simulink model "TestStructure"  (R2023b)
settings: Solver=FixedStepDiscrete  StartTime=0.0  StopTime=inf  FixedStep=SampleTime  RelTol=1e-3
InitFcn:
  | SampleTime = 0.001;
  | ButtonValue=0;
  | load("BusConfig.mat");
undefined symbols (not defined in the file): DiscIntNeverNeededParam
libraries: slrealtimeethercatlib x219, dspfdesign x28, dspstat3 x23, simulink x21, slpidlib x10, dspswit3 x8, commfilt2 x2, dspsigops x1
(part 8 of 8)

== matlab function TestStructure/InterForceControlTask/AO/ColdStartEventGate ==
  data: event_in input; event_out output; t_now input; T_base_default input
function event_out = fcn(event_in, t_now, T_base_default)
%#codegen
% Pass the first AO event immediately, then reject duplicate pulses that
% are too close to the data-derived baseline gait period.
persistent prev seen_first last_accept_t
if isempty(prev)
    prev = false;
    seen_first = false;
    last_accept_t = 0.0;
end

event_out = 0.0;
curr = (event_in ~= 0);
rise = (~prev) && curr;
prev = curr;
if ~rise
    return;
end

T = double(T_base_default);
if ~isfinite(T) || T <= 0.5 || T >= 4.0
    T = 1.66;
end
min_interval = max(0.5, 0.5 * T);
if ~seen_first || (t_now - last_accept_t) >= min_interval
    event_out = 1.0;
    seen_first = true;
    last_accept_t = t_now;
end
end

== matlab function TestStructure/InterForceControlTask/AO/Subsystem1/Abs-based selector/MATLAB Function ==
  data: candidate input; pos_env input; neg_env input; mode output
function mode = select_event_mode(candidate, pos_env, neg_env)
% mode =  1：使用正事件
% mode = -1：使用负事件
% mode =  0：切换时跳过当前目标事件

persistent current_mode pending_mode switching seen_target_event

if isempty(current_mode)
    current_mode = 1;          % 默认用正事件
    pending_mode = 1;
    switching = false;
    seen_target_event = false;
end

% 参数
ratio = 1.2;       % 正负幅值差超过20%才认为该切换
k = 0.4;           % 阈值比例，和你外面的动态阈值保持一致
th_min = 0.05;     % 最小阈值，按你的candidate量级调整

% 根据正负包络得到各自阈值
th_pos = max(k * pos_env, th_min);
th_neg = max(k * neg_env, th_min);

% 默认输出当前模式
mode = current_mode;

% 判断当前应该使用哪个事件方向
desired_mode = current_mode;

if pos_env > ratio * neg_env
    desired_mode = 1;
elseif neg_env > ratio * pos_env
    desired_mode = -1;
end

% 如果发现应该切换：只登记，不立刻切换
if ~switching && desired_mode ~= current_mode
    pending_mode = desired_mode;
    switching = true;
    seen_target_event = false;
end

% 如果正在切换，跳过目标方向的第一个事件脉冲
if switching

    if pending_mode == 1
        target_event = candidate > th_pos;
    else
        target_event = candidate < -th_neg;
    end

    % 目标方向第一个脉冲出现：跳过
    if target_event
        mode = 0;
        seen_target_event = true;
        return;
    end

    % 目标方向第一个脉冲已经结束：正式切换
    if seen_target_event && ~target_event
        current_mode = pending_mode;
        switching = false;
        seen_target_event = false;
        mode = current_mode;
        return;
    end

    % 还没等到目标事件时，继续保持旧模式
    mode = current_mode;
end

== matlab function TestStructure/InterForceControlTask/AO/Subsystem1/If Action Subsystem2/MATLAB Function1 ==
  data: u input; y output; threadhold input
function y = fcn(u, threadhold)
a = mean(u);
b = u - a;
y = (b(end) - b(1))*abs(a)*200;

if abs(y) <= threadhold
    y = 0;
end

== matlab function TestStructure/InterForceControlTask/AO2/MATLAB Function ==
  data: phi input; y output; deltaphi input
function y = fcn(phi,deltaphi)
%#codegen

a = (phi - deltaphi);

if deltaphi<0
    if(a>1)
        a = a-1;
    else
    end
else
    if(a<0)
        a = a+1;
    else
    end
end

y = a;

== matlab function TestStructure/InterForceControlTask/AO/Subsystem1/MATLAB Function ==
  data: y output; u input
function y = Decline_effective(u)
persistent d_start;
persistent d_end;
persistent d_max;

if isempty(d_start)
    d_start = 0;
    d_end = 1;
    d_max = 0;
end

y = 0;

if (u <= d_max * 0.1) && (d_end == 1)
    d_start = 1;
    d_end = 0;
end

if (d_start==1)
    if u < d_max
        y = 1;
        d_start = 0;
    else
        d_max = max(u,d_max);
    end
end

if (d_start == 0)
    if u <= d_max * 0.1
        d_max = 0;
        d_end = 1;
    end
end

== matlab function TestStructure/InterForceControlTask/TorqueController/Subsystem2/MATLAB Function ==
  data: y output; u input
function y = Decline_effective(u)
persistent d_start;
persistent d_end;
persistent d_max;

if isempty(d_start)
    d_start = 0;
    d_end = 1;
    d_max = 0;
end

y = 0;

if (u <= d_max * 0.1) && (d_end == 1)
    d_start = 1;
    d_end = 0;
end

if (d_start==1)
    if u < d_max
        y = 1;
        d_start = 0;
    else
        d_max = max(u,d_max);
    end
end

if (d_start == 0)
    if u <= d_max * 0.1
        d_max = 0;
        d_end = 1;
    end
end

== matlab function TestStructure/InterForceControlTask/AO3/MATLAB Function ==
  data: phi input; y output; deltaphi input
function y = fcn(phi,deltaphi)
%#codegen

a = (phi - deltaphi);

if deltaphi<0
    if(a>1)
        a = a-1;
    else
    end
else
    if(a<0)
        a = a+1;
    else
    end
end

y = a;

== matlab function TestStructure/InterForceControlTask/TorqueController/Subsystem2/If Action Subsystem2/MATLAB Function1 ==
  data: u input; y output; threadhold input
function y = fcn(u, threadhold)
a = mean(u);
b = u - a;
y = (b(end) - b(1))*abs(a)*200;

if abs(y) <= threadhold
    y = 0;
end

== matlab function TestStructure/InterForceControlTask/TorqueController/MATLAB Function3 ==
  data: u input; y output
function y = fcn(u)
    y = (3/(1+exp(-40*(u+(1/10))))-3)+(3/(1+exp(-40*(u-(1/10)))));
end

== matlab function TestStructure/InterForceControlTask/AO/Subsystem1/Detector1/VoltageToFootLoad ==
  data: p8 input; leftLoad output; rightLoad output
function [leftLoad, rightLoad] = VoltageToFootLoad(p8)
%#codegen
p = double(p8(:));

% The selected channels use a stable unloaded voltage across sessions.
% A fixed baseline avoids false events while a cold-start maximum settles.
baseline = 2.6 * ones(8,1);
leftIdx = int32([2 3]);
rightIdx = int32([6 7]);

load = max(baseline - p, 0.0);
for n = 1:2
    k = leftIdx(n);
    if ~isfinite(p(k)) || p(k) <= 0.1
        load(k) = 0.0;
    end
    k = rightIdx(n);
    if ~isfinite(p(k)) || p(k) <= 0.1
        load(k) = 0.0;
    end
end

leftLoad = sum(load(leftIdx));
rightLoad = sum(load(rightIdx));
end

== matlab function TestStructure/InterForceControlTask/DMP/MATLAB Function6 ==
  data: weights output; p_resampled_in input; centers output; widths output; y0 output; v0 output; goal output; segment_len input; A_demo output; y0_demo output; StartEvent input; ComputeEnable input; alpha_z input; alpha_x input; progress output; ChunkSize input; done output
function [weights, centers, widths, y0, v0, goal, A_demo, y0_demo, progress, done] = ...
    learn_from_trajectory_incremental( ...
        p_resampled_in, segment_len, StartEvent, ComputeEnable, ...
        alpha_z, alpha_x, ChunkSize)
%#codegen

% —— 统一成 double，避免上游给到单/整型 —— 
% p_resampled_in = double(p_resampled_in);
% segment_len    = double(segment_len);
% StartEvent     = double(StartEvent);
% ComputeEnable  = double(ComputeEnable);
% alpha_z        = double(alpha_z);
% alpha_x        = double(alpha_x);
% ChunkSize      = double(ChunkSize);

% —— 常量 —— 
n_bfs  = 400;
tau    = 1.0;
beta_z = alpha_z / 4.0;

% —— 持久变量（全部提前声明并默认初始化）——
persistent L idx dt_norm ...
           y0_demo_t A_demo_t y0_t v0_t goal_t ...
           centers_t widths_t ...
           num_t den_t ...
           prev_y prev_v inited ...
           p_norm_t demo_v_t demo_a_t

if isempty(inited)
    % 初始默认（保证任何路径下都有定义）
    inited     = false;
    L          = 1;
    idx        = 1;
    dt_norm    = 1.0;
    y0_demo_t  = 0.0;
    A_demo_t   = 1.0;
    y0_t       = 0.0;
    v0_t       = 0.0;
    goal_t     = 0.0;
    centers_t  = zeros(1, n_bfs);
    widths_t   = ones(1, n_bfs);
    num_t      = zeros(1, n_bfs);
    den_t      = zeros(1, n_bfs);
    prev_y     = 0.0;
    prev_v     = 0.0;
    p_norm_t   = 0.0;
    demo_v_t   = 0.0;
    demo_a_t   = 0.0;
end

% —— 输出缺省值（即使未开始也有稳定输出）——
weights  = zeros(1, n_bfs);
centers  = centers_t;
widths   = widths_t;
y0       = y0_t;
v0       = v0_t;
goal     = goal_t;
A_demo   = A_demo_t;
y0_demo  = y0_demo_t;
progress = 0.0;
done     = 0.0;

% ====== 若 StartEvent 触发：初始化一轮增量学习 ======
if (StartEvent ~= 0) && (segment_len >= 2)
    L = max(1, floor(segment_len));          % 防御性：整数长度
    % 幅值统计（整段一次，代价极小）
    % y0_demo_t = p_resampled_in(1);
    pmax = max(p_resampled_in(1:L));
    pmin = min(p_resampled_in(1:L));
    %y0_demo由pmin替代
    y0_demo_t = pmin;
    A_demo_t = pmax - pmin;
    if A_demo_t < 1e-8, A_demo_t = 1.0; end
    
    p_norm_t  = (p_resampled_in(1:L) - pmin) / A_demo_t;
    y0_t   = p_norm_t(1);
    goal_t = p_norm_t(L);

    dt_norm = tau / max(1, (L - 1));
    if L >= 2
        demo_v_t       = [ (p_norm_t(2)-p_norm_t(1))/dt_norm ; diff(p_norm_t)./dt_norm ];
        demo_a_t       = [ (demo_v_t(2)-demo_v_t(1))/dt_norm ; diff(demo_v_t)./dt_norm ];
        v0_t           = demo_v_t(1);
    else
        demo_v_t = 0.0;  demo_a_t = 0.0;  v0_t = 0.0;
    end
    
    % 基函数网格
    % ext = 4;
    cc  = exp(-alpha_x * linspace(0, 1, n_bfs));
    ww  = n_bfs^2 ./ cc;
    centers_t = cc;
    widths_t  = ww;

    % % 基函数网格（首尾各裁4）
    % ext = 4;
    % cc  = exp(-alpha_x * linspace(0, 1, n_bfs + 2*ext));
    % ww  = (n_bfs + 2*ext)^2 ./ cc;
    % centers_t = cc((1+ext):(end-ext));
    % widths_t  = ww((1+ext):(end-ext));

    % 累加器清零与指针
    num_t = zeros(1, n_bfs);
    den_t = zeros(1, n_bfs);
    idx   = 1;
    prev_y = y0_t; 
    prev_v = v0_t;

    inited = true;
end

% —— 若尚未开始（没收到 StartEvent），直接返回缺省输出 —— 
if ~inited
    return;
end

% ====== 1ms Tick：每次吃 ChunkSize 个样本 ======
if (ComputeEnable ~= 0) && (idx <= L)
    % 夹紧 ChunkSize 合理范围
    cs = min( max(1, floor(ChunkSize)), L - idx + 1 );

    for k = 0:(cs-1)
        j  = idx + k;                      % 第 j 个样本（1-based）

        % —— 用持久的预计算序列 —— 
        yj = p_norm_t(j);
        vj = demo_v_t(j);
        aj = demo_a_t(j);

        prev_y = yj; 
        prev_v = vj;

        % 规范时间与门控
        tj = (j - 1) * dt_norm;
        sj = exp(-alpha_x * tj);

        % f_target（知乎改进方案）
        f_target = ( tau*tau*aj - alpha_z*(beta_z*(goal_t - yj) - tau*vj) )/alpha_z ...
                   + sj*(goal_t - y0_t);
        % f_target = ( tau*tau*aj - alpha_z*(beta_z*(goal_t - yj) - tau*vj) )/alpha_z;

        % 累加充要统计量
        psi_row = exp( - widths_t .* (sj - centers_t).^2 );
        num_t   = num_t + (sj * f_target) * psi_row;
        den_t   = den_t + (sj*sj) * psi_row;
    end
    idx = idx + cs;
end

% —— 进度条 —— 
progress = min(1.0, idx / max(1, L));

% ====== 全段完成：输出权重并置 done ======
if idx > L
    weights = num_t ./ (den_t + 1e-12);
    centers = centers_t;
    widths  = widths_t;
    y0      = y0_t;
    v0      = v0_t;
    goal    = goal_t;
    A_demo  = A_demo_t;
    y0_demo = y0_demo_t;

    done    = 1.0;
    % 如需下一次 StartEvent 重新开始，可在此处选择：
    % inited = false;
end
end

== matlab function TestStructure/InterForceControlTask/AO2/Select/MATLAB Function1 ==
  data: u input; y output
function y = fcn(u)
    y = (3/(1+exp(-40*(u+(1/10))))-3)+(3/(1+exp(-40*(u-(1/10)))));
end

== matlab function TestStructure/InterForceControlTask/AO2/Subsystem/Subsystem/MATLAB Function ==
  data: phi input; y output; deltaphi input
function y = fcn(phi,deltaphi)
%#codegen

a = floor(phi/(2*pi));

y = (phi - a*2*pi -deltaphi*pi);

== matlab function TestStructure/InterForceControlTask/AO2/Subsystem/Subsystem1/MATLAB Function ==
  data: phi input; y output; deltaphi input
function y = fcn(phi,deltaphi)
%#codegen

a = floor(phi/(2*pi));

y = (phi - a*2*pi -deltaphi*pi);

== matlab function TestStructure/InterForceControlTask/AO2/Subsystem/Subsystem3/MATLAB Function ==
  data: phi input; y output; deltaphi input
function y = fcn(phi,deltaphi)
%#codegen

a = floor(phi/(2*pi));

y = (phi - a*2*pi -deltaphi*pi);

== matlab function TestStructure/InterForceControlTask/AO2/Subsystem/Subsystem5/MATLAB Function ==
  data: phi input; y output; deltaphi input
function y = fcn(phi,deltaphi)
%#codegen

a = floor(phi/(2*pi));

y = (phi - a*2*pi -deltaphi*pi);

== matlab function TestStructure/InterForceControlTask/DMP/MATLAB Function8 ==
  data: FastStartEvent input; weights input; centers input; widths input; y0 input size=[1 1]; v0 input; goal input size=[1 1]; A_demo input size=[1 1]; y0_demo input size=[1 1]; alpha_z input; alpha_x input; TriggerEvent input; s input size=[1 1]; dt input size=[1 1]; tau input size=[1 1]; y_real output; Amplitude input; HoldRatio input; HoldRefSec input; v_real output; right_start_real input; playback_phi output
function [y_real,v_real,playback_phi] = trajectory_generator( ...
    FastStartEvent, weights, centers, widths, y0, v0, goal, A_demo, y0_demo, ...
    alpha_z, alpha_x, TriggerEvent, s, dt, tau, Amplitude, ...
    HoldRatio, HoldRefSec, right_start_real )
% 生成端（残差版）：支持 tau 时间缩放 + 完成后 hold + min–max 反归一化
% 输入 s：这里把它当作 AO 的“相位”Phi∈[0,1] 来用（线性锯齿即可）
% 输出 y_real：反归一化后的轨迹（y*A_demo + pmin），其中 y0_demo 端口承载 pmin
%#codegen

% --- 常量 ---
beta_z = alpha_z / 4.0;
SAFE_CENTER = 0.0;   % 不稳定时希望缓慢回到的"安全角度"，单位与 y_real 一致，可改
SAFE_BAND   = 0.0;   % 认为"已经够安全”的带宽，比如 ±5 度内就直接原地 hold
ENABLE_STABLE_GATE = false;   % true=启用稳定门，false=关闭稳定门

% --- 持久状态（内部 y, y_dot；相位缩放用的内部进度 u；完成标志） ---
persistent y y_dot u phi_prev inited trig_prev fast_prev fast_seen_count dmp_ready_for_start started pending_reset just_started first_playback_protected
persistent hold_ticks hold_active
persistent delay_ticks delay_active prev_y_real prev_v_real refrac_ticks prestart_hold prestart_hold_valid  
persistent A_prev y0d_prev
persistent g_tAcc g_buf g_has g_outOK g_safeY

if isempty(refrac_ticks), refrac_ticks = 0; end
if isempty(fast_prev), fast_prev = 0.0; end
if isempty(fast_seen_count), fast_seen_count = int32(0); end
if isempty(dmp_ready_for_start), dmp_ready_for_start = 0.0; end
if isempty(first_playback_protected), first_playback_protected = false; end
if isempty(A_prev),   A_prev   = A_demo; end
if isempty(y0d_prev), y0d_prev = y0_demo; end



if isempty(prev_y_real), prev_y_real = 0; end
if isempty(prestart_hold), prestart_hold = 0.0; end
if isempty(prestart_hold_valid), prestart_hold_valid = false; end
if isempty(prev_v_real), prev_v_real = 0; end

if isempty(inited)
    first_cycle = true;
    y = y0;
    y_dot = v0;
    u = 0;  
    phi_prev = 0;
    finished = false;
    trig_prev = false;
    inited = true;
    started = false;
    pending_reset = false;   % 新增：检测到开始沿后，下一帧再复位
    just_started  = false;   % 新增：复位后的首帧只打起点，不推进
    y0_latch = y0; v0_latch = v0; goal_latch = goal;   % 参数锁存（用于握手）
    hold_ticks = 0;
    hold_active = false;
    delay_ticks = 0;
    delay_active = false;
    eps_param = 1e-6;
    g_tAcc = 0.0;              % 距上次沿累计的时间
    g_buf  = [Inf Inf Inf];    % 最近3个周期（秒）
    g_has  = 0;                % 已记录周期数(<=3)
    g_outOK = ~ENABLE_STABLE_GATE;           % 是否允许输出
    g_safeY = 0.0;              % 不稳定时要渐近回到的安全位(这里取0)
end

playback_phi = u;
y_real = prev_y_real;   % 默认保持上一帧
v_real = prev_v_real;

% --- 相位增量（把第 11 个输入 s 当作相位 Phi）---
Phi = s;
raw_dphi = Phi - phi_prev;   % 保留原始差分用于回绕沿判定
dphi = raw_dphi;
% 处理 1→0 回绕；防止偶发负跳
if dphi < -0.5
    dphi = (1 - phi_prev) + Phi;
elseif dphi < 0
    dphi = 0;
end
wrap_edge = (raw_dphi < -0.5);  % 新增：相位 1->0 回绕沿
phi_prev = Phi;

% --- Phase0Event 上升沿检测 ---
trig_edge = false;

if (trig_prev == false && TriggerEvent == true)
    trig_edge = true;
end
trig_prev = TriggerEvent;

fast_curr = (FastStartEvent ~= 0);
fast_edge_raw = ((fast_prev == 0.0) && fast_curr);
fast_prev = double(fast_curr);
fast_edge = fast_edge_raw;
if fast_edge_raw
    fast_seen_count = fast_seen_count + 1;
end

% ===== 稳定门：用 TriggerEvent 的上升沿统计周期 =====
if ENABLE_STABLE_GATE
    % 累计时间
    g_tAcc = g_tAcc + dt;

    if trig_edge
        T = g_tAcc;         % 一个完整周期（秒）
        g_tAcc = 0.0;

        % 只保留最近3个周期
        g_buf = [g_buf(2:3) T];
        g_has = min(g_has + 1, 3);

        % 判稳：max-min <= max(绝对阈, 相对阈*均值)
        if g_has >= 3
            Tmean   = (g_buf(1)+g_buf(2)+g_buf(3))/3;
            Tspan   = max(g_buf) - min(g_buf);
            TOL_REL = 0.40;
            TOL_ABS = 0.20;
            g_outOK = (Tspan <= max(TOL_ABS, TOL_REL*Tmean));
        else
            g_outOK = false;
        end
    end
else
    g_outOK = true;
end
% ===== 稳定门 END =====


% ---------- DMP ready 前：不推进、不积分，输出当前右腿位置 ----------
if ~started
    % The first FastStart already means one complete trajectory window
    % has been learned. Take over immediately at this boundary.
    start_edge = fast_edge;
else
    start_edge = false;
    if trig_edge
        start_edge = true;
    end
end

if ~started
    if start_edge
        started = true;
        first_playback_protected = true;
        dmp_ready_for_start = 0.0;
        first_cycle = false;
        pending_reset = false;
        just_started = false;
        y0_latch = y0; v0_latch = v0; goal_latch = goal;
        A_seed = sign(A_demo) * max(abs(A_demo), 1e-9);


        y = (right_start_real - y0_demo) / A_seed;
        y_dot = 0;
        u = 0;
        finished = false;
        A_prev = A_seed;
        y0d_prev = y0_demo;
        y_real = right_start_real;
        v_real = 0;
        prev_y_real = y_real;
        prev_v_real = v_real;
        g_safeY = y_real;
        return;
    else
        y_real = right_start_real;
        v_real = 0;
        prev_y_real = y_real;
        prev_v_real = v_real;
        g_safeY = y_real;
        return;
    end
end
% ---------- 以上仅影响“第一拍开始前/开始当拍”；之后流程不变 ----------

% ---- 开始后的第1帧：真正用已更新的 y0/v0 执行复位，并返回 ----
if pending_reset

    % ====== 软复位 + 坐标重投影（无跳变、无扭动）======
    % 新一拍的仿射参数（可能刚换）
    A_new   = A_demo;
    y0_new  = y0_demo;

    % 防除零
    A_new = sign(A_new) * max(abs(A_new), 1e-9);
    A_prev = sign(A_prev) * max(abs(A_prev), 1e-9);

    % 1) 位置连续：把内部 y 重写为“在新坐标下仍等于上一帧输出”的值
    %    令 y_new 满足：prev_y_real = y_new * A_new + y0_new
    y = (prev_y_real - y0_new) / A_new;

    % 2) 速度连续（可选但强烈建议）：让 y_real_dot 连续
    %    之前：y_real_dot_prev = y_dot * A_prev
    %    之后：y_real_dot_now  = y_dot_new * A_new  → 令两者相等
    y_dot = y_dot * (A_prev / A_new);

    % 3) 开启新拍：只把进度清零，其它状态保持
    u             = 0;
    finished      = false;
    pending_reset = false;

    % 4) 更新“上一拍参数”备下次用
    A_prev   = A_new;
    y0d_prev = y0_new;

    % % 5) 当帧输出保持不变（绝对连续）
    % y_real      = prev_y_real;
    % prev_y_real = y_real;
    % v_real = prev_v_real;
    % prev_v_real = v_real;
    % return;

end

% ---- 开始后的第2帧：只输出起点，不推进、不积分 ----
if just_started
    y_real = y0 * A_demo + y0_demo;

    % ---- 稳定器输出门控 + 回到0附近 ----
    if g_outOK
        % 稳定：直接用 DMP 输出，并同步安全位
        g_safeY = y_real;
    else
        % 不稳定：不跟 DMP，缓慢回到0附近
        T_back = 0.3;                         % 回零时间常数(秒)，可调
        alpha  = dt / max(T_back, 1e-3);
        if alpha > 1, alpha = 1; end
        if abs(g_safeY - SAFE_CENTER) <= SAFE_BAND
            % 已在安全带内：直接 hold，不再往 SAFE_CENTER 拉
            y_real = g_safeY;
        else
            % 不在安全带：缓慢向 SAFE_CENTER 收敛
            g_safeY = g_safeY + alpha * (SAFE_CENTER - g_safeY);
            y_real  = g_safeY;
        end
    end
    v_real      = 0;
    prev_y_real = y_real;  % 保证后续复位/重投影的连续性
    prev_v_real = v_real;
    return;
end


% === 新增：首播 hold 段（保持 y0，冻结积分与u推进）===
if hold_active
    if hold_ticks > 0
        hold_ticks = hold_ticks - 1;
        % 输出固定起点；不更新 u / y_dot / y
        y_real = y * A_demo + y0_demo;
        v_real = y_dot * A_demo;
        prev_v_real = v_real;
        return;
    else
        hold_active = false;    % hold 结束，开始正常推进
        end
end

% 是否允许未完成就抢占（true=保持原行为；false=等当前拍走完）
allow_preempt = true;  % 建议设 false 来保幅值/保形状

if (trig_edge && refrac_ticks==0)
    if allow_preempt || (u >= 1 - 1e-6)
        % 允许抢占，或当前拍已完成：照常进入延迟/复位流程

        delay_ticks  = max(0, round((HoldRatio * HoldRefSec) / max(dt,1e-6)));
        delay_active = (delay_ticks > 0);
        pending_reset = true; 
        finished = false; 
        first_cycle = false;
        refrac_ticks  = round(0.02 / max(dt,1e-6));
        % if delay_active
        %     y_real = prev_y_real; 
        %     prev_y_real = y_real; 
        %     v_real = 0;
        %     prev_v_real = v_real;
        %     return;
        % else
        %     pending_reset = true; 
        %     y_real = prev_y_real; 
        %     prev_y_real = y_real; 
        %     v_real = 0;
        %     prev_v_real = v_real;
        %     return;
        % end
    else
        % 不允许抢占且未完成：忽略这次触发，继续把当前拍播完
        % （也可以在这里置一个 overrun 标志供你观察）
        % y_real 默认已经是 prev_y_real；继续向下正常生成
    end
end


% === 延迟阶段：保持上一拍末值，直到 delay_ticks 归零 ===
if delay_active
    if delay_ticks > 0
        delay_ticks = delay_ticks - 1;
        y_real       = prev_y_real;
        v_real       = prev_v_real;
        prev_y_real  = y_real;
        prev_v_real  = v_real;
        return;
    else
        delay_active = false;
        % pending_reset = true;                          % 标记下一帧在 pending_reset 中复位
        % y_real = prev_y_real;                          % 这一帧仍保持末值
        % v_real = 0;
        % prev_v_real = v_real;
        % return;
    end
end

% ====== 拍中参数变化的“连续重投影”（无跳变、无扭动）======
% 任何时候只要 A_demo 或 y0_demo 发生明显变化，就把内部 y/y_dot
% 映射到新坐标，使 y_real 与其导数连续，再继续积分。
eps_aff = 1e-9;  % 防除零
A_now   = sign(A_demo) * max(abs(A_demo), eps_aff);
A_old   = sign(A_prev) * max(abs(A_prev), eps_aff);

if (abs(A_now - A_prev) > 1e-6) || (abs(y0_demo - y0d_prev) > 1e-6)
    % 1) 位置连续：令 y_new 满足 prev_y_real = y_new*A_now + y0_demo
    y = (prev_y_real - y0_demo) / A_now;

    % 2) 速度连续：y_real_dot 旧= y_dot*A_old，新= y_dot_new*A_now → 相等
    y_dot = y_dot * (A_old / A_now);

    % 3) 更新“上一帧参数”
    A_prev   = A_now;
    y0d_prev = y0_demo;

    % 4) 当帧保持输出（绝对连续），下一帧再按新坐标继续积分
    y_real      = prev_y_real;
    prev_y_real = y_real;
    v_real = prev_v_real;
    prev_v_real = v_real;
    return;
end




% --- 内部进度按 tau 缩放推进（时间放缩）---
u = u + dt / max(tau, 1e-6);     % standard DMP scaling; delayed events only prevent early reset
if u > 1
    u = 1;
elseif u < 0
    u = 0;
end

% --- 若已完成：强制 hold 在终点并直接反归一化输出 ---
if u >= 1 - 1e-6
    first_playback_protected = false;
    finished = true;

    % 当前 DMP 的“原始”位置/速度
    y_dmp = y * A_demo + y0_demo;
    v_dmp = A_demo * y_dot;

    if g_outOK
        % —— 稳定：直接跟随 DMP —— 
        y_real  = y_dmp;
        v_real  = v_dmp;
        g_safeY = y_real;
    else
        % —— 不稳定：按 SAFE_CENTER 慢慢回零，同时给出和该轨迹一致的速度 —— 
        T_back = 0.3;
        alpha  = dt / max(T_back, 1e-3);
        if alpha > 1, alpha = 1; end

        if abs(g_safeY - SAFE_CENTER) <= SAFE_BAND
            % 已在安全带内：原地 hold
            y_new = g_safeY;
        else
            % 不在安全带：缓慢向 SAFE_CENTER 收敛
            g_safeY = g_safeY + alpha * (SAFE_CENTER - g_safeY);
            y_new  = g_safeY;
        end

        y_real = y_new;
        % 用输出位置的一阶差分作为“安全”的参考速度
        v_real = (y_new - prev_y_real) / max(dt, 1e-6);
    end

    prev_y_real = y_real;
    prev_v_real = v_real;
    return;
end


% --- 门控/相位：与学习端保持一致（线性或指数二选一） ---
% 线性门控（推荐）：ss 从 1→0
% ss = 1 - u;
% if ss < 1e-6, ss = 1e-6; end

% 指数门控
ss = exp(-alpha_x * u);

% --- 基函数响应（在 s 空间计算；此处用 ss 作为 s）---
psi = exp( - widths .* (ss - centers).^2 );
den = sum(psi) + 1e-12;
if den == 0
    % 极端数值保护
    psi(1) = 1; den = 1;
end
f_shape = (psi * weights.') / den;

% 残差版：f 再乘 s（=ss），仅拟合“形状残差”
f = f_shape * ss;

% --- 动力学（残差版配对：保留 -alpha_z*ss*(goal-y0)）---
y_ddot = ( alpha_z*(beta_z*(goal - y) - tau*y_dot) ...
           + alpha_z * f * Amplitude ...
           - alpha_z * ss * (goal - y0) ) / (tau^2);

% --- 数值积分 ---
y_dot = y_dot + dt * y_ddot;
y     = y     + dt * y_dot;

% --- 反归一化（学习端为 min–max：p_norm=(p - pmin)/A_demo）---
% 因此生成端对应 y_real = y*A_demo + pmin；这里 y0_demo 端口承载 pmin

y_real = y * A_demo + y0_demo;
v_real = A_demo * y_dot;

% --- 反归一化后，先保存 DMP 的“原始”位置和速度 ---
y_dmp = y * A_demo + y0_demo;
v_dmp = A_demo * y_dot;

if g_outOK
    % ======= 稳定：直接用 DMP 的位置和速度 =======
    y_real  = y_dmp;
    v_real  = v_dmp;
    g_safeY = y_real;
else
    % ======= 不稳定：只跟稳定器的缓慢回零轨迹 =======
    T_back = 0.3;                            
    alpha  = dt / max(T_back, 1e-3);
    if alpha > 1, alpha = 1; end

    if abs(g_safeY - SAFE_CENTER) <= SAFE_BAND
        % 已在安全带内：原地 hold
        y_new = g_safeY;
    else
        % 不在安全带：缓慢向 SAFE_CENTER 收敛
        g_safeY = g_safeY + alpha * (SAFE_CENTER - g_safeY);
        y_new  = g_safeY;
    end

    y_real = y_new;
    % 用稳定器轨迹的一阶差分当作参考速度
    v_real = (y_new - prev_y_real) / max(dt, 1e-6);
end

prev_y_real = y_real;
prev_v_real = v_real;


if refrac_ticks > 0
    refrac_ticks = refrac_ticks - 1;
end
end

== matlab function TestStructure/InterForceControlTask/DMP/Phase_shifter ==
  data: Phase0Event_H input; t_ref output; t_now input; T_base_default input
function t_ref = DelayAfterTwoEvents_tref(Phase0Event_H, t_now, T_base_default)
%#codegen
% The data-derived default is active immediately. After three measured
% raw AO periods, switch to the rolling three-period average.
persistent prev seen_first t_prev T1 T2 T3 measured_count t_ref_last
if isempty(prev)
    default_T = sanitizePeriod(T_base_default);
    prev = false;
    seen_first = false;
    t_prev = 0.0;
    T1 = default_T;
    T2 = default_T;
    T3 = default_T;
    measured_count = int32(0);
    t_ref_last = default_T;
end

t_ref = t_ref_last;
curr = (Phase0Event_H ~= 0);
rise = (~prev) && curr;
prev = curr;

if rise
    if ~seen_first
        seen_first = true;
        t_prev = t_now;
    else
        dt = t_now - t_prev;
        if isfinite(dt) && dt > 0.5 && dt < 4.0
            T3 = T2;
            T2 = T1;
            T1 = dt;
            measured_count = measured_count + 1;
            if measured_count >= 3
                t_ref_last = (T1 + T2 + T3) / 3.0;
            end
        end
        t_prev = t_now;
    end
end
t_ref = t_ref_last;
end

function T = sanitizePeriod(value)
T = double(value);
if ~isfinite(T) || T <= 0.5 || T >= 4.0
    T = 1.66;
end
end

== matlab function TestStructure/InterForceControlTask/DMP/Subsystem/DelaySamplesFromPrev ==
  data: t_prev input; ratio input; N output; dt input
function N = DelaySamplesFromPrev(t_prev, ratio, dt)
%#codegen
% 按上一拍周期 t_prev 和当前 ratio 计算整数采样延迟，
% 但一拍内保持不变

persistent N_hold t_prev_last inited
if isempty(inited)
    inited     = false;
    N_hold     = int32(0);
    t_prev_last= 0.0;
end

dt    = max(dt,1e-6);
t_prev= max(t_prev,5*dt);
ratio = max(ratio,0.0);

%  只在检测到 t_prev 发生变化时，更新一次 N_hold
%   （即：每次 AO 识别到新的周期，才换一个延迟）
if ~inited || abs(t_prev - t_prev_last) > 0.5*dt
    Nd        = round((ratio * t_prev) / dt);    % 整数采样
    N_hold    = int32(max(0, Nd));
    t_prev_last = t_prev;
    inited    = true;
end

% 一拍内输出始终为 N_hold（ratio 中途再变也不影响当前拍）
N = N_hold;

== matlab function TestStructure/InterForceControlTask/DMP/Subsystem/EventDelay ==
  data: trig_in input; N input; out output; tau input
function out = PhaseEventDelay_ScaledIntervals(trig_in, N, tau)
%#codegen
% N is valid from cold startup because Phase_shifter starts from the
% data-derived baseline. Queue the first delayed candidate immediately.
MAX_QUEUE = int32(128);
persistent prev sample_idx last_candidate have_candidate scaled_target
persistent queue head tail count
if isempty(prev)
    prev = false;
    sample_idx = int64(0);
    last_candidate = int64(0);
    have_candidate = false;
    scaled_target = int64(0);
    queue = zeros(1, 128, 'int64');
    head = int32(1);
    tail = int32(1);
    count = int32(0);
end

tau = max(double(tau), 1e-6);
out = false;
curr = (trig_in ~= 0);
edge = (~prev) && curr;
prev = curr;

if edge
    candidate = sample_idx + int64(max(0, round(double(N))));
    if ~have_candidate
        scaled_target = candidate;
        have_candidate = true;
    else
        candidate_period = candidate - last_candidate;
        if candidate_period > 0
            scaled_target = scaled_target + int64(max(1, round(tau * double(candidate_period))));
        end
    end
    last_candidate = candidate;

    if scaled_target > 0 && count < MAX_QUEUE
        queue(tail) = scaled_target;
        tail = tail + 1;
        if tail > MAX_QUEUE, tail = int32(1); end
        count = count + 1;
    end
end

if count > 0 && sample_idx >= queue(head)
    out = true;
    head = head + 1;
    if head > MAX_QUEUE, head = int32(1); end
    count = count - 1;
end
sample_idx = sample_idx + 1;
end

== matlab function TestStructure/InterForceControlTask/AO1/MATLAB Function ==
  data: phi input; y output; deltaphi input
function y = fcn(phi,deltaphi)
%#codegen

a = (phi - deltaphi);

if deltaphi<0
    if(a>1)
        a = a-1;
    else
    end
else
    if(a<0)
        a = a+1;
    else
    end
end

y = a;

== matlab function TestStructure/InterForceControlTask/DMP/Subsystem/PhiOmega_DelayRebuild ==
  data: event_delay input; dt_sec input; phi_delay output; omega_delay output; T_base_default input
function [phi_delay, omega_delay] = RebuildPhiOmegaFromDelayedEvent(event_delay, dt_sec, T_base_default)
%#codegen
% Diagnostic delayed-event phase. Hold the shared default until three
% complete delayed periods exist.
persistent prev_evt t_since T1 T2 T3 T_avg measured_count seen_first
if isempty(prev_evt)
    default_T = sanitizePeriod(T_base_default);
    prev_evt = false;
    t_since = 0.0;
    T1 = default_T;
    T2 = default_T;
    T3 = default_T;
    T_avg = default_T;
    measured_count = int32(0);
    seen_first = false;
end

dt_sec = max(dt_sec, 1e-6);
curr = (event_delay ~= 0);
rise = (~prev_evt) && curr;
prev_evt = curr;
t_since = t_since + dt_sec;

if rise
    if seen_first
        last_period = t_since;
        if isfinite(last_period) && last_period > 0.5 && last_period < 6.0
            T3 = T2;
            T2 = T1;
            T1 = last_period;
            measured_count = measured_count + 1;
            if measured_count >= 3
                T_avg = (T1 + T2 + T3) / 3.0;
            end
        end
    else
        seen_first = true;
    end
    t_since = 0.0;
end

omega_delay = 1.0 / max(T_avg, 0.1);
phi_delay = min(max(t_since * omega_delay, 0.0), 1.0);
end

function T = sanitizePeriod(value)
T = double(value);
if ~isfinite(T) || T <= 0.5 || T >= 4.0
    T = 1.66;
end
end

== matlab function TestStructure/InterForceControlTask/DMP/compute_chunk ==
  data: segment_len input; cs output; T_prev input; tick_s input
function cs = compute_chunk(segment_len, T_prev, tick_s)
%#codegen
% 计算每个1ms tick应处理的样本数（ChunkSize）
% 保证输出 cs 为 double，避免 uint16 → double 的隐式写入错误

% 明确输出类型（初始化一次即可设定为 double）
cs = 0.0;

% 转 double，防止上游给了 uint16/int
segment_len_d = double(segment_len);
T_prev_d      = double(T_prev);
tick_d        = double(tick_s);

% 防御性处理
if ~(isfinite(segment_len_d) && segment_len_d > 0)
    segment_len_d = 1.0;
end
if ~(isfinite(T_prev_d) && T_prev_d > 0)
    % 第一拍没有上一周期长度时给个保守默认
    T_prev_d = 0.8;   % 例如默认0.8s步期，可按需修改
end
tick_d = max(tick_d, 1e-6);

% 计算 M 和 ChunkSize
M  = max(1.0, round(T_prev_d / tick_d));
cs = ceil(segment_len_d / M);
cs = min(max(cs, 1.0), segment_len_d);
end

== matlab function TestStructure/InterForceControlTask/DMP/compute_chunk2 ==
  data: phase_edge input; N_available output; start_edge input; compute_tick input; done input; N_used output; Slack output
function [N_available, N_used, Slack] = tick_counters(phase_edge, start_edge, compute_tick, done)
%#codegen
persistent cnt_cycle cnt_used latched_used have_used
if isempty(cnt_cycle)
    cnt_cycle = 0; cnt_used = 0; latched_used = 0; have_used = false;
end

% 周期计数：Phase0Event 上升沿复位
if phase_edge ~= 0
    N_available = cnt_cycle;     % 上一拍统计值
    Slack       = max(0, N_available - latched_used);
    cnt_cycle   = 0;             % 开始新一拍
else
    N_available = -1;            % 非更新时刻可输出 -1 或保持上次外部 Sample&Hold
    Slack       = -1;
end

% 一拍内的 10ms 窗口统计
if compute_tick ~= 0
    cnt_cycle = cnt_cycle + 1;
end

% 学习用的 10ms 计数：从 start_edge 后开始累加，直到 done
if start_edge ~= 0
    cnt_used = 0; have_used = false;
end
if (compute_tick ~= 0) && (done == 0)
    cnt_used = cnt_used + 1;
end
if (done ~= 0) && ~have_used
    latched_used = cnt_used;     % 只锁存一次
    have_used = true;
end

% 输出 N_used（锁存值）
N_used = latched_used;
end

== matlab function TestStructure/InterForceControlTask/AO3/PhaseCorrection/MATLAB Function ==
  data: t_t_start input; Omega output; u input; phi output
function [Omega, phi] = fcn(t_t_start, u)
    % t_t_start: 秒表时间（当前这一步走了多久）
    % u: 复位脉冲（Peaks）
    
    % 声明持久化变量，记住最近 3 步的时间和上一时刻的数据
    persistent T1 T2 T3 T_avg_held prev_t prev_u
    
    % 开机初始化：默认周期 1.66 秒 (约等于 0.6 步频)
    if isempty(T1)
        T1 = 1.66; 
        T2 = 1.66;
        T3 = 1.66;
        T_avg_held = 1.66;
        prev_t = 0;
        prev_u = 0;
    end
    
    % 检测复位信号 u 的上升沿 (从 0 变 1 的瞬间)
    if u > 0.5 && prev_u <= 0.5
        
        % 使用 prev_t (脉冲来临前一瞬间的最大累积时间) 作为这一步的真实用时
        current_T = prev_t;
        
        % 步态合理性保护 (0.5秒到4秒之间算有效步数)
        if current_T > 0.5 && current_T < 4.0
            T3 = T2;
            T2 = T1;
            T1 = current_T;
            
            % 算出最近 3 步平均时间
            T_avg_held = (T1 + T2 + T3) / 3; 
        end
    end
    
    % 记忆当前数值，留给下个周期对比
    prev_t = t_t_start;
    prev_u = u;
    
    % --- 输出 1: Omega ---
    if T_avg_held > 0.1
        Omega = 1 / T_avg_held;
    else
        Omega = 0;
    end
    
    % --- 输出 2: Phi ---
    % 核心魔法：当前时间除以平均总时间，直接算出完美的 0~1.0 相位！
    % 因为 t_t_start 在波谷时会突变为 0，所以 phi 也会瞬间产生完美的 1.0->0 跌落！
    raw_phi = t_t_start * Omega; 

    % 如果步子迈得太久，phi 就停在 1.0 处"悬停等待"
    phi = min(raw_phi, 1.0);
end

== matlab function TestStructure/InterForceControlTask/AO3/PhaseCorrection/MATLAB Function1 ==
  data: raw_peak input; valid_peak output; t input
function valid_peak = Gait_Stabilizer(raw_peak, t)
    % raw_peak: 前端传来的完美瞬时脉冲
    % t: 仿真时间
    
    % 只需要记住三个东西：上次踩下的时间、上一步花了多久、当前是否稳定
    persistent last_peak_t T_prev is_stable
    
    if isempty(last_peak_t)
        last_peak_t = -10.0;
        T_prev = 0;
        is_stable = 0; % 默认：未稳定，冷眼旁观
    end
    
    valid_peak = 0; % 默认不输出
    
    % 【超时检测】：如果你突然停下来超过 2.5 秒没走
    % 系统立刻判定“失去稳态”，把大门关上，等你重新找回节奏
    if (t - last_peak_t) > 2.5
        is_stable = 0; 
    end
    
    % 当一个完美的物理脉冲到来时：
    if raw_peak > 0.5 
        
        % 算一下这一步花了多久
        T_curr = t - last_peak_t;
        
        % 过滤掉极度不合理的跨步（比如小于0.6秒的纯噪点，或大于2.5秒的停顿）
        if T_curr > 0.6 && T_curr < 2.5
            
            % 【核心稳态判定】：
            % 如果这一步的时间，跟上一步的时间，误差小于 0.2 秒！
            if abs(T_curr - T_prev) < 0.2
                is_stable = 1; % 节奏对上了！判定为稳态！
            else
                is_stable = 0; % 节奏断了（比如深一脚浅一脚），打回未稳定状态！
            end
            
            % 更新记忆，留给下一步对比
            T_prev = T_curr; 
        end
        
        % 【终极放行】：只有当系统处于“稳态”时，才把这个脉冲吐给下游！
        if is_stable == 1
            valid_peak = 1;
        end
        
        last_peak_t = t; % 无论稳不稳定，都要记录这次物理脉冲发生的时间
    end
end

== matlab function TestStructure/InterForceControlTask/AO3/Select/MATLAB Function1 ==
  data: u input; y output
function y = fcn(u)
    y = (3/(1+exp(-40*(u+(1/10))))-3)+(3/(1+exp(-40*(u-(1/10)))));
end

== matlab function TestStructure/InterForceControlTask/AO3/Subsystem/Subsystem/MATLAB Function ==
  data: phi input; y output; deltaphi input
function y = fcn(phi,deltaphi)
%#codegen

a = floor(phi/(2*pi));

y = (phi - a*2*pi -deltaphi*pi);

== matlab function TestStructure/InterForceControlTask/AO3/Subsystem/Subsystem1/MATLAB Function ==
  data: phi input; y output; deltaphi input
function y = fcn(phi,deltaphi)
%#codegen

a = floor(phi/(2*pi));

y = (phi - a*2*pi -deltaphi*pi);

== matlab function TestStructure/InterForceControlTask/AO3/Subsystem/Subsystem3/MATLAB Function ==
  data: phi input; y output; deltaphi input
function y = fcn(phi,deltaphi)
%#codegen

a = floor(phi/(2*pi));

y = (phi - a*2*pi -deltaphi*pi);

== matlab function TestStructure/InterForceControlTask/AO3/Subsystem/Subsystem5/MATLAB Function ==
  data: phi input; y output; deltaphi input
function y = fcn(phi,deltaphi)
%#codegen

a = floor(phi/(2*pi));

y = (phi - a*2*pi -deltaphi*pi);

== matlab function TestStructure/InterForceControlTask/TorqueController/MATLAB Function1 ==
  data: raw_peak input; valid_peak output; t input
function valid_peak = Gait_Stabilizer(raw_peak, t)
    % raw_peak: 前端传来的完美瞬时脉冲
    % t: 仿真时间
    
    % 上次踩下的时间、上一步花了多久、当前是否稳定
    persistent last_peak_t T_prev is_stable
    
    if isempty(last_peak_t)
        last_peak_t = -10.0;
        T_prev = 0;
        is_stable = 0; % 默认：未稳定
    end
    
    valid_peak = 0; % 默认不输出
    
    % 突然停下来超过 2.5 秒没走
    % 系统立刻判定“失去稳态”，把大门关上，等你重新找回节奏
    if (t - last_peak_t) > 2.5
        is_stable = 0; 
    end
    
    % 当一个完美的物理脉冲到来时：
    if raw_peak > 0.5 
        
        % 算一下这一步花了多久
        T_curr = t - last_peak_t;
        
        % 过滤掉极度不合理的跨步（比如小于0.6秒的纯噪点，或大于2.5秒的停顿）
        if T_curr > 0.6 && T_curr < 2.5
            
            % 如果这一步的时间，跟上一步的时间，误差小于 0.2 秒
            if abs(T_curr - T_prev) < 0.2
                is_stable = 1; 
            else
                is_stable = 0; 
            end
            
            % 更新记忆，留给下一步对比
            T_prev = T_curr; 
        end
        
        if is_stable == 1
            valid_peak = 1;
        end
        
        last_peak_t = t; % 无论稳不稳定，都要记录这次物理脉冲发生的时间
    end
end

== matlab function TestStructure/InterForceControlTask/TorqueController2/MATLAB Function ==
  data: valid_peak input; actual_torque output; target_torque input; t input; current_gain output
function [actual_torque, current_gain] = Torque_Manager(valid_peak, target_torque, t)
    % valid_peak: 右腿脉冲
    % target_torque: 底层PD控制器算出来的原始力矩 
    % t: 当前系统时间 (Clock 模块接入)
    
    persistent step_count last_peak_t prev_peak
    
    if isempty(step_count)
        step_count = 0;
        last_peak_t = -10.0;
        prev_peak = 0;
    end
    
    % 1. 抓取迈步信号，更新步数和秒表
    if valid_peak > 0.5 && prev_peak <= 0.5
        step_count = step_count + 1;
        last_peak_t = t;
    end
    prev_peak = valid_peak;
    
    % 2. 基础缓入增益：前5步慢慢给力
    base_gain = min(step_count / 5.0, 1.0);
    
    % 3. 停步安全检测与快速淡出
    time_since_last = t - last_peak_t;
    fade_gain = 1.0; % 默认不打折
    
    % 假设正常走一步最多 1.5 秒
    if time_since_last > 2.0
        % 停步超过 2.0 秒：切断动力
        fade_gain = 0;
        
        % 既然停下了，步数也清零，下次起步重新慢慢缓入
        if time_since_last > 3.0
            step_count = 0; 
            base_gain = 0;
        end
        
    elseif time_since_last > 1.5
        % 1.5秒到 2.0秒之间：执行 0.5 秒的平滑卸力
        % 比如 1.5秒时 gain=1.0，2.0秒时 gain=0.0，线性下降
        fade_gain = (2.0 - time_since_last) * 2.0; 
    end
    
    % 4. 最终
    final_gain = base_gain * fade_gain;
    
    % 只有 gain 大于 0，力矩才能放行
    actual_torque = target_torque * final_gain;
    
    % 输出当前的总增益
    current_gain = final_gain; 
end

== matlab function TestStructure/InterForceControlTask/TorqueController2/MATLAB Function1 ==
  data: raw_peak input; valid_peak output; t input
function valid_peak = Gait_Stabilizer(raw_peak, t)
    % raw_peak: 前端传来的完美瞬时脉冲
    % t: 仿真时间
    
    % 上次踩下的时间、上一步花了多久、当前是否稳定
    persistent last_peak_t T_prev is_stable
    
    if isempty(last_peak_t)
        last_peak_t = -10.0;
        T_prev = 0;
        is_stable = 0; % 默认：未稳定
    end
    
    valid_peak = 0; % 默认不输出
    
    % 突然停下来超过 2.5 秒没走
    % 系统立刻判定“失去稳态”，把大门关上，等你重新找回节奏
    if (t - last_peak_t) > 2.5
        is_stable = 0; 
    end
    
    % 当一个完美的物理脉冲到来时：
    if raw_peak > 0.5 
        
        % 算一下这一步花了多久
        T_curr = t - last_peak_t;
        
        % 过滤掉极度不合理的跨步（比如小于0.6秒的纯噪点，或大于2.5秒的停顿）
        if T_curr > 0.6 && T_curr < 2.5
            
            % 如果这一步的时间，跟上一步的时间，误差小于 0.2 秒
            if abs(T_curr - T_prev) < 0.2
                is_stable = 1; 
            else
                is_stable = 0; 
            end
            
            % 更新记忆，留给下一步对比
            T_prev = T_curr; 
        end
        
        if is_stable == 1
            valid_peak = 1;
        end
        
        last_peak_t = t; % 无论稳不稳定，都要记录这次物理脉冲发生的时间
    end
end

== matlab function TestStructure/InterForceControlTask/TorqueController2/MATLAB Function2 ==
  data: valid_peak input; total_steps output
function total_steps = Step_Counter(valid_peak)
    % 只需记住当前的累计步数，和上次脉冲的状态（用来抓上升沿）
    persistent count prev_peak
    
    if isempty(count)
        count = 0;       % 开机步数为 0
        prev_peak = 0;
    end
    
    % 只有在完美脉冲抬头的瞬间，步数才 +1
    if valid_peak > 0.5 && prev_peak <= 0.5
        count = count + 1;
    end
    
    % 更新记忆，输出当前总步数
    prev_peak = valid_peak;
    total_steps = count;
end

== matlab function TestStructure/InterForceControlTask/AO1/PhaseCorrection/MATLAB Function ==
  data: t_t_start input; Omega output; u input; phi output
function [Omega, phi] = fcn(t_t_start, u)
    % t_t_start: 秒表时间（当前这一步走了多久）
    % u: 复位脉冲（Peaks）
    
    % 声明持久化变量，记住最近 3 步的时间和上一时刻的数据
    persistent T1 T2 T3 T_avg_held prev_t prev_u
    
    % 开机初始化：默认周期 1.66 秒 (约等于 0.6 步频)
    if isempty(T1)
        T1 = 1.66; 
        T2 = 1.66;
        T3 = 1.66;
        T_avg_held = 1.66;
        prev_t = 0;
        prev_u = 0;
    end
    
    % 检测复位信号 u 的上升沿 (从 0 变 1 的瞬间)
    if u > 0.5 && prev_u <= 0.5
        
        % 使用 prev_t (脉冲来临前一瞬间的最大累积时间) 作为这一步的真实用时
        current_T = prev_t;
        
        % 步态合理性保护 (0.5秒到4秒之间算有效步数)
        if current_T > 0.5 && current_T < 4.0
            T3 = T2;
            T2 = T1;
            T1 = current_T;
            
            % 算出最近 3 步平均时间
            T_avg_held = (T1 + T2 + T3) / 3; 
        end
    end
    
    % 记忆当前数值，留给下个周期对比
    prev_t = t_t_start;
    prev_u = u;
    
    % --- 输出 1: Omega ---
    if T_avg_held > 0.1
        Omega = 1 / T_avg_held;
    else
        Omega = 0;
    end
    
    % --- 输出 2: Phi ---
    % 当前时间除以平均总时间，直接算出完美的 0~1.0 相位！
    % 因为 t_t_start 在波谷时会突变为 0，phi 也会产生1.0->0 跌落
    raw_phi = t_t_start * Omega; 

    % 迈得太久，phi 就停在 1.0
    phi = min(raw_phi, 1.0);
end

== matlab function TestStructure/InterForceControlTask/AO1/PhaseCorrection/MATLAB Function1 ==
  data: raw_peak input; valid_peak output; t input
function valid_peak = Gait_Stabilizer(raw_peak, t)
    % raw_peak: 前端传来的完美瞬时脉冲
    % t: 仿真时间
    
    % 上次踩下的时间、上一步花了多久、当前是否稳定
    persistent last_peak_t T_prev is_stable
    
    if isempty(last_peak_t)
        last_peak_t = -10.0;
        T_prev = 0;
        is_stable = 0; % 默认：未稳定，冷眼旁观
    end
    
    valid_peak = 0; % 默认不输出
    
    % 突然停下来超过 2.5 秒没走
    % 系统立刻判定“失去稳态”，把大门关上，等你重新找回节奏
    if (t - last_peak_t) > 2.5
        is_stable = 0; 
    end
    
    % 当一个完美的物理脉冲到来时：
    if raw_peak > 0.5 
        
        % 算一下这一步花了多久
        T_curr = t - last_peak_t;
        
        % 过滤掉极度不合理的跨步（比如小于0.6秒的纯噪点，或大于2.5秒的停顿）
        if T_curr > 0.6 && T_curr < 2.5
            
            % 如果这一步的时间，跟上一步的时间，误差小于 0.2 秒
            if abs(T_curr - T_prev) < 0.2
                is_stable = 1; 
            else
                is_stable = 0; 
            end
            
            % 更新记忆，留给下一步对比
            T_prev = T_curr; 
        end
        
        if is_stable == 1
            valid_peak = 1;
        end
        
        last_peak_t = t; % 无论稳不稳定，都要记录这次物理脉冲发生的时间
    end
end

== matlab function TestStructure/InterForceControlTask/AO1/PhaseCorrection/MATLAB Function2 ==
  data: valid_peak input; total_steps output
function total_steps = Step_Counter(valid_peak)
    % 只需记住当前的累计步数，和上次脉冲的状态（用来抓上升沿）
    persistent count prev_peak
    
    if isempty(count)
        count = 0;       % 开机步数为 0
        prev_peak = 0;
    end
    
    % 只有在完美脉冲抬头的瞬间，步数才 +1
    if valid_peak > 0.5 && prev_peak <= 0.5
        count = count + 1;
    end
    
    % 更新记忆，输出当前总步数
    prev_peak = valid_peak;
    total_steps = count;
end

== matlab function TestStructure/Robot/MotorPositonInit1/MATLAB Function1 ==
  data: P input; y output; t input
function y  = fcn(P, t)
y = P(1)*t^5+P(2)*t^4+P(3)*t^3+P(4)*t^2+P(5)*t+P(6);

== matlab function TestStructure/InterForceControlTask/AO1/Select/MATLAB Function1 ==
  data: u input; y output
function y = fcn(u)
    y = (3/(1+exp(-40*(u+(1/10))))-3)+(3/(1+exp(-40*(u-(1/10)))));
end

== matlab function TestStructure/Robot/MotorPositonInit1/MATLAB Function2 ==
  data: P input; y output; t input
function y  = fcn(P, t)
y = P(1)*t^5+P(2)*t^4+P(3)*t^3+P(4)*t^2+P(5)*t+P(6);

== matlab function TestStructure/InterForceControlTask/AO1/Subsystem/Subsystem/MATLAB Function ==
  data: phi input; y output; deltaphi input
function y = fcn(phi,deltaphi)
%#codegen

a = floor(phi/(2*pi));

y = (phi - a*2*pi -deltaphi*pi);

== matlab function TestStructure/InterForceControlTask/AO1/Subsystem/Subsystem1/MATLAB Function ==
  data: phi input; y output; deltaphi input
function y = fcn(phi,deltaphi)
%#codegen

a = floor(phi/(2*pi));

y = (phi - a*2*pi -deltaphi*pi);

== matlab function TestStructure/InterForceControlTask/AO1/Subsystem/Subsystem3/MATLAB Function ==
  data: phi input; y output; deltaphi input
function y = fcn(phi,deltaphi)
%#codegen

a = floor(phi/(2*pi));

y = (phi - a*2*pi -deltaphi*pi);

== matlab function TestStructure/InterForceControlTask/AO1/Subsystem/Subsystem5/MATLAB Function ==
  data: phi input; y output; deltaphi input
function y = fcn(phi,deltaphi)
%#codegen

a = floor(phi/(2*pi));

y = (phi - a*2*pi -deltaphi*pi);

== matlab function TestStructure/InterForceControlTask/TorqueController/MATLAB Function2 ==
  data: valid_peak input; total_steps output
function total_steps = Step_Counter(valid_peak)
    % 只需记住当前的累计步数，和上次脉冲的状态（用来抓上升沿）
    persistent count prev_peak
    
    if isempty(count)
        count = 0;       % 开机步数为 0
        prev_peak = 0;
    end
    
    % 只有在完美脉冲抬头的瞬间，步数才 +1
    if valid_peak > 0.5 && prev_peak <= 0.5
        count = count + 1;
    end
    
    % 更新记忆，输出当前总步数
    prev_peak = valid_peak;
    total_steps = count;
end

== matlab function TestStructure/InterForceControlTask/AO/MATLAB Function ==
  data: phi input; y output; deltaphi input
function y = fcn(phi,deltaphi)
%#codegen

a = (phi - deltaphi);

if deltaphi<0
    if(a>1)
        a = a-1;
    else
    end
else
    if(a<0)
        a = a+1;
    else
    end
end

y = a;

== matlab function TestStructure/InterForceControlTask/TorqueController/Subsystem2/Buffer Function ==
  data: u input; y output
function y = Buffer(u)
%#codegen
persistent buf

if isempty(buf)
    buf = zeros(30,1);
end

buf(1:29) = buf(2:30);
buf(30) = u;

y = buf;

== matlab function TestStructure/Robot/MotorPositonInit1/MATLAB Function3 ==
  data: P input; y output; t input
function y  = fcn(P, t)
y = P(1)*t^5+P(2)*t^4+P(3)*t^3+P(4)*t^2+P(5)*t+P(6);

== matlab function TestStructure/Robot/MotorPositonInit1/MATLAB Function4 ==
  data: P input; y output; t input
function y  = fcn(P, t)
y = P(1)*t^5+P(2)*t^4+P(3)*t^3+P(4)*t^2+P(5)*t+P(6);
